simulink library "posAugCoef_cl"  (R2022a)
settings: Solver=VariableStepAuto  StartTime=0.0  StopTime=10.0  RelTol=1e-3
undefined symbols (not defined in the file): aRoll, aYaw, azuSweep, bandGap, bRoll, bYaw, DiscIntNeverNeededParam, elevSet, elevStart, env, fftSwitch, FLIGHTCONTROLLER, fltCtrl, fltCtrlPath, FREQ, hiGainTime, initializeBussesFromBlock, intSat, K_filt, lockTime, orientExitTime, orientLaps, pathEstimCtrl, pathLaps, pthCtrl1, rollAmp, rollFreq, rollPhase, rollPow, thetaIGain, thetaPGain, vhcl, yawAmp, yawFreq, yawPhase
libraries: dspsigops x10, slpidlib x5, firstOrderFilter_ul x3, velocityAngle_ul x2, pathFollowingCtrlAoATurb_cl x1, pathFollowingCtrlAoATurbCoef_cl x1, courseFollowLookAhead_cl x1, ctrlAllocMatrix3CompCoef_cl x1, eulAng2RotMat_ul x1, angleBtw2Vecs_ul x1, vrlib x1, alphaBeta_ul x1
(part 2 of 2)

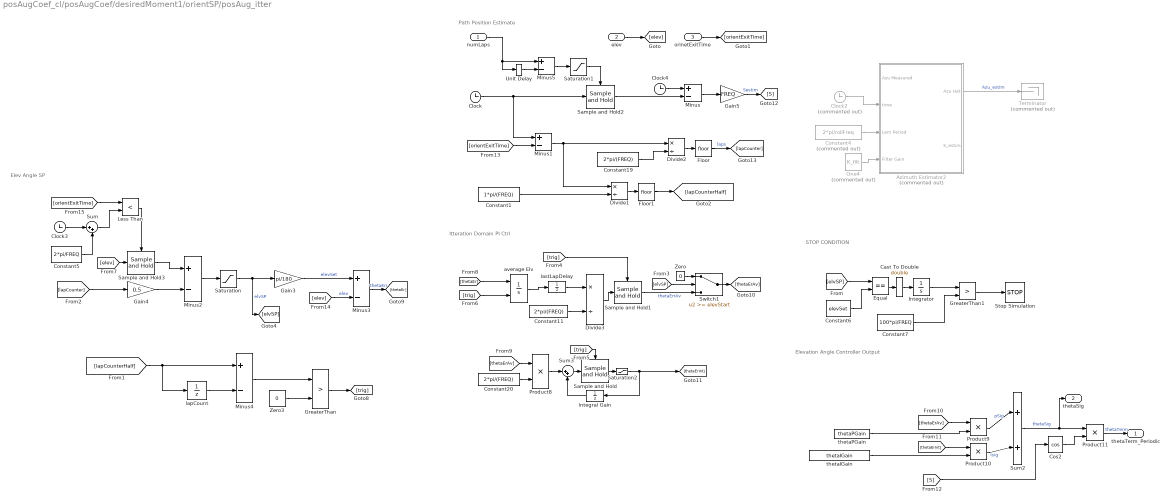
== system posAugCoef_cl/posAugCoef/desiredMoment1/orientSP/posAug_itter ==
  note: STOP CONDITION
  note: Elev Angle SP
  note: Itteration Domain PI Ctrl
  note: Path Position Estimate
  note: Elevation Angle Controller Output
  numLaps : Inport
  elev : Inport  Port=2
  orinetExitTime : Inport  Port=3
  Azimuth Estimator2 : Subsystem  Commented=on
  Cast To Double : DataTypeConversion  OutDataTypeStr=double  SaturateOnIntegerOverflow=off  RndMeth=Floor
  Clock : Clock
  Clock2 : Clock  Commented=on
  Clock3 : Clock
  Clock4 : Clock
  Constant1 : Constant  Value=1*pi/(FREQ)
  Constant11 : Constant  Value=2*pi/(FREQ)
  Constant19 : Constant  Value=2*pi/(FREQ)
  Constant20 : Constant  Value=2*pi/(FREQ)
  Constant4 : Constant  Commented=on  Value=2*pi/rollFreq
  Constant5 : Constant  Value=2*pi/FREQ
  Constant6 : Constant  Value=elevSet
  Constant7 : Constant  Value=100*pi/FREQ
  Cos2 : Trigonometry  Operator=cos
  Divide1 : Product  Inputs=*/
  Divide2 : Product  Inputs=*/
  Divide3 : Product  Inputs=*/
  Equal : RelationalOperator  Operator===  OutDataTypeStr=boolean  RndMeth=Simplest  InputSameDT=off
  Floor : Rounding
  Floor1 : Rounding
  Gain3 : Gain  Gain=pi/180
  Gain4 : Gain  Gain=0.5
  Gain5 : Gain  Gain=FREQ
  GreaterThan : RelationalOperator  Operator=>  OutDataTypeStr=boolean  RndMeth=Simplest  InputSameDT=off
  GreaterThan1 : RelationalOperator  Operator=>  OutDataTypeStr=boolean  RndMeth=Simplest  InputSameDT=off
  Integrator : Integrator
  Less Than : RelationalOperator  Operator=<  OutDataTypeStr=boolean  RndMeth=Simplest  InputSameDT=off
  Minus{,1..5} (6 alike) : Sum  Inputs=+-
  One4 : Constant  Commented=on  Value=K_filt  OutDataTypeStr=Inherit: Inherit via back propagation
  Product{8..11} (4 alike) : Product
  Sample and Hold : dspsigops/Sample and Hold  trig=Rising edge  initCond=0  latchinput=off
  Sample and Hold1 : dspsigops/Sample and Hold  trig=Rising edge  initCond=0  latchinput=off
  Sample and Hold2 : dspsigops/Sample and Hold  trig=Rising edge  initCond=0  latchinput=off
  Sample and Hold3 : dspsigops/Sample and Hold  trig=Rising edge  initCond=elevSet  latchinput=off
  Saturation : Saturate  UpperLimit=elevSet+15  LowerLimit=elevSet
  Saturation1 : Saturate  UpperLimit=pathLaps  LowerLimit=0
  Saturation2 : Saturate  UpperLimit=200  LowerLimit=-200
  Stop Simulation : Stop
  Sum : Sum  Inputs=|++
  Sum2 : Sum  Inputs=|++
  Sum3 : Sum  Inputs=|++
  Switch1 : Switch  Threshold=elevStart  SaturateOnIntegerOverflow=off  InputSameDT=off
  Terminator : Terminator  Commented=on
  Unit Delay : UnitDelay  SampleTime=-1  HasFrameUpgradeWarning=on
  Zero : Constant  Value=0  OutDataTypeStr=Inherit: Inherit via back propagation
  Zero3 : Constant  Value=0  OutDataTypeStr=Inherit: Inherit via back propagation
  average Elv : Integrator  ExternalReset=rising
  integral Gain : UnitDelay  SampleTime=-1  HasFrameUpgradeWarning=on
  lapCount : UnitDelay  SampleTime=-1  HasFrameUpgradeWarning=on
  lastLapDelay : UnitDelay  SampleTime=-1  HasFrameUpgradeWarning=on
  thetaIGain : Constant  Value=thetaIGain
  thetaPGain : Constant  Value=thetaPGain
  thetaTerm_Periodic : Outport
  thetaSig : Outport  Port=2
  wires:
  Sum2/1 -> thetaSig/1, Product11/1  "thetaSig"
  [thetaErAv] -> Product8/1
  lapCount/1 -> Minus4/2
  thetaIGain/1 -> Product10/2
  Product11/1 -> thetaTerm_Periodic/1  "thetaTerm"
  GreaterThan/1 -> [trig]
  thetaPGain/1 -> Product9/2
  [trig] -> average Elv/2
  [thetaErInt] -> Product10/1
  [elev] -> Minus3/2  "elev"
  average Elv/1 -> lastLapDelay/1
  Divide2/1 -> Floor/1
  Zero3/1 -> GreaterThan/2
  Floor/1 -> [lapCounter]  "laps"
  Product10/1 -> Sum2/2  "Isig"
  Product9/1 -> Sum2/1  "pSig"
  Cos2/1 -> Product11/2
  Saturation2/1 -> [thetaErInt], integral Gain/1
  Sample and Hold1/1 -> Switch1/3  "thetaErrAv"
  Product8/1 -> Sum3/1
  [trig] -> Sample and Hold1/Trigger
  [thetaErAv] -> Product9/1
  Constant20/1 -> Product8/2
  Sample and Hold/1 -> Saturation2/1
  integral Gain/1 -> Sum3/2
  Minus1/1 -> Divide1/1, Divide2/1
  Divide3/1 -> Sample and Hold1/1
  Saturation/1 -> [elvSP], Gain3/1  "elvSP"
  Constant11/1 -> Divide3/2
  Gain5/1 -> [S]  "Sestim"
  [trig] -> Sample and Hold/Trigger
  lastLapDelay/1 -> Divide3/1
  Minus3/1 -> [thetaEr]  "thetaErr"
  Minus4/1 -> GreaterThan/1
  [thetaEr] -> average Elv/1
  Sum3/1 -> Sample and Hold/1
  Constant19/1 -> Divide2/2
  Clock/1 -> Minus1/1, Sample and Hold2/1
  elev/1 -> [elev]
  Divide1/1 -> Floor1/1
  Floor1/1 -> [lapCounterHalf]
  Constant1/1 -> Divide1/2
  [lapCounter] -> Gain4/1
  Sample and Hold3/1 -> Minus2/1
  Minus2/1 -> Saturation/1
  Gain3/1 -> Minus3/1  "elevSet"
  numLaps/1 -> Unit Delay/1, Minus5/1
  Unit Delay/1 -> Minus5/2
  [elvSP] -> Switch1/2
  Zero/1 -> Switch1/1
  Switch1/1 -> [thetaErAv]
  Gain4/1 -> Minus2/2
  [orientExitTime] -> Minus1/2
  [lapCounterHalf] -> lapCount/1, Minus4/1
  Constant4/1 -> Azimuth Estimator2/3(Lem Period)
  Clock2/1 -> Azimuth Estimator2/2(time)
  Azimuth Estimator2/1(Azu Hat) -> Terminator/1  "Azu_estim"
  One4/1 -> Azimuth Estimator2/4(Filter Gain)
  [S] -> Cos2/1
  Minus5/1 -> Saturation1/1
  Saturation1/1 -> Sample and Hold2/Trigger
  Clock4/1 -> Minus/1
  [elvSP] -> Equal/1
  Equal/1 -> Cast To Double/1
  Constant6/1 -> Equal/2
  Integrator/1 -> GreaterThan1/1
  Constant7/1 -> GreaterThan1/2
  GreaterThan1/1 -> Stop Simulation/1
  Cast To Double/1 -> Integrator/1
  Minus/1 -> Gain5/1
  [orientExitTime] -> Less Than/1
  Sum/1 -> Less Than/2
  Clock3/1 -> Sum/1
  Constant5/1 -> Sum/2
  Less Than/1 -> Sample and Hold3/Trigger
  [elev] -> Sample and Hold3/1
  orinetExitTime/1 -> [orientExitTime]
  Sample and Hold2/1 -> Minus/2

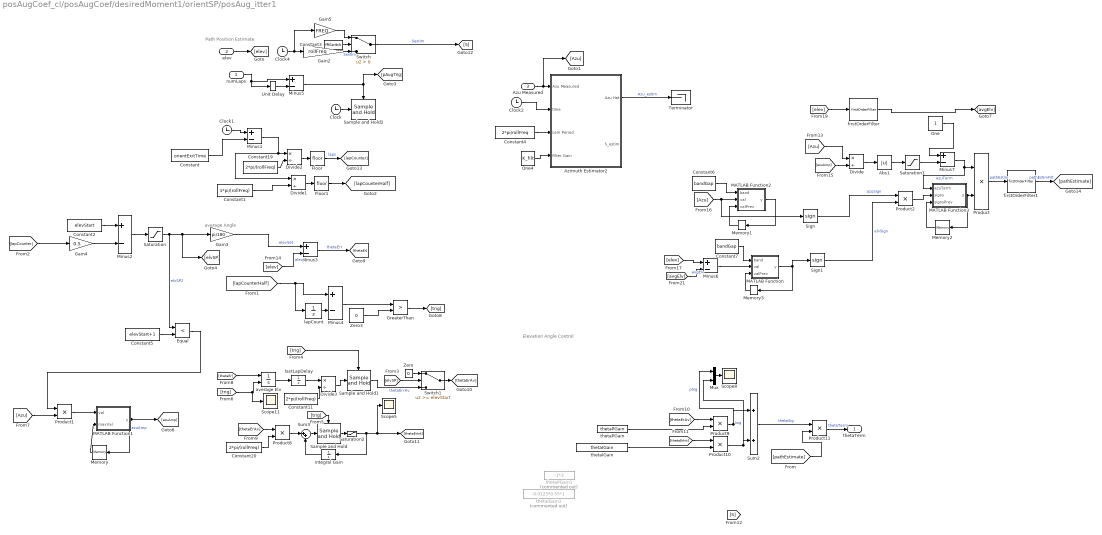
== system posAugCoef_cl/posAugCoef/desiredMoment1/orientSP/posAug_itter1 ==
  note: average Angle
  note: Path Position Estimate
  note: Elevation Angle Control
  numLaps : Inport
  elev : Inport  Port=2
  Azu Measured : Inport  Port=3
  Abs1 : Abs  SaturateOnIntegerOverflow=off
  Azimuth Estimator2 : Subsystem
  Clock{,1..2,4} (4 alike) : Clock
  Constant : Constant  Value=orientExitTime
  Constant1 : Constant  Value=1*pi/(rollFreq)
  Constant11 : Constant  Value=2*pi/(rollFreq)
  Constant19 : Constant  Value=2*pi/(rollFreq)
  Constant2 : Constant  Value=elevStart
  Constant20 : Constant  Value=2*pi/(rollFreq)
  Constant3 : Constant  Value=fftSwitch
  Constant4 : Constant  Value=2*pi/rollFreq
  Constant5 : Constant  Value=elevStart+1
  Constant6 : Constant  Value=bandGap
  Constant7 : Constant  Value=bandGap
  Divide{,1..3} (4 alike) : Product  Inputs=*/
  Equal : RelationalOperator  Operator=<  OutDataTypeStr=boolean  RndMeth=Simplest  InputSameDT=off
  Floor : Rounding
  Floor1 : Rounding
  Gain2 : Gain  Gain=rollFreq
  Gain3 : Gain  Gain=pi/180
  Gain4 : Gain  Gain=0.5
  Gain5 : Gain  Gain=FREQ
  GreaterThan : RelationalOperator  Operator=>  OutDataTypeStr=boolean  RndMeth=Simplest  InputSameDT=off
  MATLAB Function : MATLAB Function  TreatAsAtomicUnit=on
  MATLAB Function1 : MATLAB Function  TreatAsAtomicUnit=on
  MATLAB Function2 : MATLAB Function  TreatAsAtomicUnit=on
  MATLAB Function3 : MATLAB Function  TreatAsAtomicUnit=on
  Memory{,1..3} (4 alike) : Memory
  Minus{1..7} (7 alike) : Sum  Inputs=+-
  Mux : Mux  Inputs=2
  One : Constant  OutDataTypeStr=Inherit: Inherit via back propagation
  One4 : Constant  Value=K_filt  OutDataTypeStr=Inherit: Inherit via back propagation
  Product{,1..2,8..11} (7 alike) : Product
  Sample and Hold : dspsigops/Sample and Hold  trig=Rising edge  initCond=0  latchinput=off
  Sample and Hold1 : dspsigops/Sample and Hold  trig=Rising edge  initCond=0  latchinput=off
  Sample and Hold2 : dspsigops/Sample and Hold  trig=Rising edge  initCond=0  latchinput=off
  Saturation : Saturate  UpperLimit=elevSet+5  LowerLimit=elevSet
  Saturation1 : Saturate  UpperLimit=1  LowerLimit=-1
  Saturation2 : Saturate  UpperLimit=intSat  LowerLimit=-intSat
  Scope11 : Scope
  Scope5 : Scope
  Scope8 : Scope
  Sign : Signum
  Sign1 : Signum
  Sum2 : Sum  Inputs=|++
  Sum3 : Sum  Inputs=|++
  Switch : Switch  Criteria=u2 > Threshold  SaturateOnIntegerOverflow=off  InputSameDT=off
  Switch1 : Switch  Threshold=elevStart  SaturateOnIntegerOverflow=off  InputSameDT=off
  Terminator : Terminator
  Unit Delay : UnitDelay  SampleTime=-1  HasFrameUpgradeWarning=on
  Zero : Constant  Value=0  OutDataTypeStr=Inherit: Inherit via back propagation
  Zero3 : Constant  Value=0  OutDataTypeStr=Inherit: Inherit via back propagation
  average Elv : Integrator  ExternalReset=rising
  firstOrderFilter : firstOrderFilter_ul/firstOrderFilter  tau=elvFilt  ic=0
  firstOrderFilter1 : firstOrderFilter_ul/firstOrderFilter  tau=pathEstimFilt  ic=0
  integral Gain : UnitDelay  SampleTime=-1  HasFrameUpgradeWarning=on
  lapCount : UnitDelay  SampleTime=-1  HasFrameUpgradeWarning=on
  lastLapDelay : UnitDelay  SampleTime=-1  HasFrameUpgradeWarning=on
  thetaIGain : Constant  Value=thetaIGain
  thetaIGain1 : Constant  Commented=on  Value=-0.0125*0.55*1
  thetaPGain : Constant  Value=thetaPGain
  thetaPGain1 : Constant  Commented=on  Value=-1*3
  thetaTerm : Outport
  wires:
  Sum2/1 -> Product11/1  "thetaSig"
  [thetaErAv] -> Product8/1
  lapCount/1 -> Minus4/2
  thetaIGain/1 -> Product10/2
  Product11/1 -> thetaTerm/1  "thetaTerm"
  GreaterThan/1 -> [trig]
  thetaPGain/1 -> Product9/2
  [trig] -> Scope11/1, average Elv/2
  [thetaErInt] -> Product10/1
  [elev] -> Minus3/2  "elev"
  average Elv/1 -> lastLapDelay/1
  Divide2/1 -> Floor/1
  Zero3/1 -> GreaterThan/2
  Floor/1 -> [lapCounter]  "laps"
  Product10/1 -> Mux/2, Sum2/2  "Isig"
  Mux/1 -> Scope8/1
  Product9/1 -> Mux/1, Sum2/1  "pSig"
  Saturation2/1 -> Scope5/1, [thetaErInt], integral Gain/1
  Sample and Hold1/1 -> Switch1/3  "thetaErrAv"
  Product8/1 -> Sum3/1
  [trig] -> Sample and Hold1/Trigger
  [thetaErAv] -> Product9/1
  Constant20/1 -> Product8/2
  Sample and Hold/1 -> Saturation2/1
  integral Gain/1 -> Sum3/2
  Minus1/1 -> Divide1/1, Divide2/1
  Divide3/1 -> Sample and Hold1/1
  Clock4/1 -> Gain5/1, Gain2/1
  Saturation/1 -> Equal/1, [elvSP], Gain3/1  "elvSP2"
  Constant11/1 -> Divide3/2
  Switch/1 -> [S]  "Sestim"
  [trig] -> Sample and Hold/Trigger
  lastLapDelay/1 -> Divide3/1
  Minus3/1 -> [thetaEr]  "thetaErr"
  Minus4/1 -> GreaterThan/1
  [thetaEr] -> average Elv/1
  Sum3/1 -> Sample and Hold/1
  Constant19/1 -> Divide2/2
  Clock1/1 -> Minus1/1
  elev/1 -> [elev]
  Minus5/1 -> [pAugTrig], Sample and Hold2/Trigger
  Clock/1 -> Sample and Hold2/1
  Divide1/1 -> Floor1/1
  Floor1/1 -> [lapCounterHalf]
  Constant1/1 -> Divide1/2
  [lapCounter] -> Gain4/1
  Constant2/1 -> Minus2/1
  Minus2/1 -> Saturation/1
  Gain3/1 -> Minus3/1  "elevSet"
  numLaps/1 -> Unit Delay/1, Minus5/1
  Unit Delay/1 -> Minus5/2
  [elvSP] -> Switch1/2
  Zero/1 -> Switch1/1
  Switch1/1 -> [thetaErAv]
  Gain4/1 -> Minus2/2
  Constant/1 -> Minus1/2
  [lapCounterHalf] -> lapCount/1, Minus4/1
  Constant3/1 -> Switch/2
  Gain2/1 -> Switch/3  "Sestim"
  Gain5/1 -> Switch/1
  Constant4/1 -> Azimuth Estimator2/3(Lem Period)
  Clock2/1 -> Azimuth Estimator2/2(time)
  Azimuth Estimator2/1(Azu Hat) -> Terminator/1  "Azu_estim"
  One4/1 -> Azimuth Estimator2/4(Filter Gain)
  Azu Measured/1 -> [Azu], Azimuth Estimator2/1(Azu Measured)
  Equal/1 -> Product1/1
  Memory/1 -> MATLAB Function1/2(maxVal)
  Product1/1 -> MATLAB Function1/1(val)
  MATLAB Function1/1(y) -> Memory/1, [azuAmp]  "azuAmp"
  Constant5/1 -> Equal/2
  [Azu] -> Product1/2
  Memory2/1 -> MATLAB Function3/3(signsPrev)
  MATLAB Function3/1(y) -> Memory2/1, Product/2
  Sign1/1 -> Product2/2  "elvSign"
  [Azu] -> Sign/1, MATLAB Function2/2(val)
  MATLAB Function/1(y) -> Memory3/1, Sign1/1
  [elev] -> Minus6/1
  Abs1/1 -> Saturation1/1
  firstOrderFilter1/1 -> [pathEstimate]  "pathEstimFilt"
  Minus7/1 -> MATLAB Function3/1(azuTerm), Product/1  "azuTerm"
  Memory3/1 -> MATLAB Function/3(valPrev)
  One/1 -> Minus7/1
  [elev] -> firstOrderFilter/1
  Constant6/1 -> MATLAB Function2/1(band)
  Product/1 -> firstOrderFilter1/1  "pathEstim"
  Saturation1/1 -> Minus7/2
  firstOrderFilter/1 -> [avgElv]
  Constant7/1 -> MATLAB Function/1(band)
  MATLAB Function2/1(y) -> Memory1/1
  Minus6/1 -> MATLAB Function/2(val)
  Sign/1 -> Product2/1  "azuSign"
  Memory1/1 -> MATLAB Function2/3(valPrev)
  [Azu] -> Divide/1
  [avgElv] -> Minus6/2  "avgElv"
  Divide/1 -> Abs1/1
  Product2/1 -> MATLAB Function3/2(signs)
  [azuAmp] -> Divide/2
  [pathEstimate] -> Product11/2

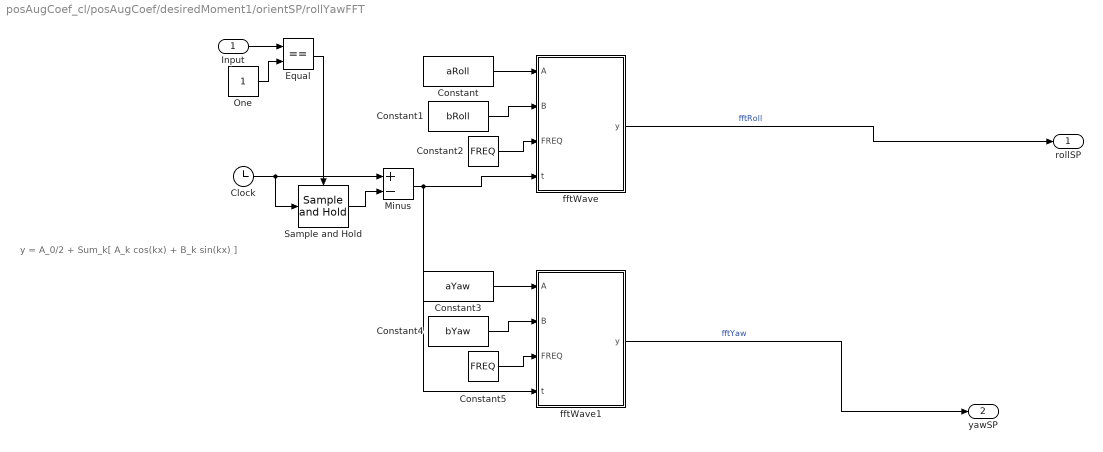
== system posAugCoef_cl/posAugCoef/desiredMoment1/orientSP/rollYawFFT ==
  note: y = A_0/2 + Sum_k[ A_k cos(kx) + B_k sin(kx) ]
  Input : Inport
  Clock : Clock
  Constant : Constant  Value=aRoll
  Constant1 : Constant  Value=bRoll
  Constant2 : Constant  Value=FREQ
  Constant3 : Constant  Value=aYaw
  Constant4 : Constant  Value=bYaw
  Constant5 : Constant  Value=FREQ
  Equal : RelationalOperator  Operator===  OutDataTypeStr=boolean  RndMeth=Simplest  InputSameDT=off
  Minus : Sum  Inputs=+-
  One : Constant  OutDataTypeStr=Inherit: Inherit via back propagation
  Sample and Hold : dspsigops/Sample and Hold  trig=Rising edge  initCond=0  latchinput=off
  fftWave : MATLAB Function  TreatAsAtomicUnit=on
  fftWave1 : MATLAB Function  TreatAsAtomicUnit=on
  rollSP : Outport
  yawSP : Outport  Port=2
  wires:
  Constant2/1 -> fftWave/3(FREQ)
  Constant1/1 -> fftWave/2(B)
  Constant/1 -> fftWave/1(A)
  Constant4/1 -> fftWave1/2(B)
  Constant5/1 -> fftWave1/3(FREQ)
  Constant3/1 -> fftWave1/1(A)
  Minus/1 -> fftWave/4(t), fftWave1/4(t)
  fftWave1/1(y) -> yawSP/1  "fftYaw"
  fftWave/1(y) -> rollSP/1  "fftRoll"
  Input/1 -> Equal/1
  One/1 -> Equal/2
  Equal/1 -> Sample and Hold/Trigger
  Clock/1 -> Minus/1, Sample and Hold/1
  Sample and Hold/1 -> Minus/2

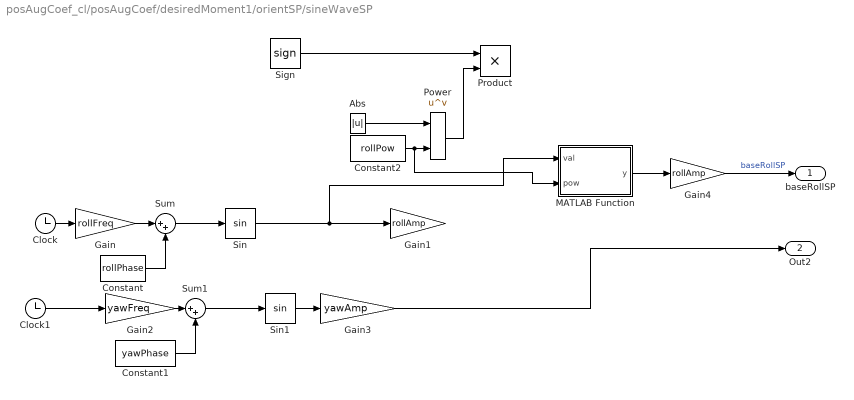
== system posAugCoef_cl/posAugCoef/desiredMoment1/orientSP/sineWaveSP ==
  Abs : Abs  SaturateOnIntegerOverflow=off
  Clock : Clock
  Clock1 : Clock
  Constant : Constant  Value=rollPhase
  Constant1 : Constant  Value=yawPhase
  Constant2 : Constant  Value=rollPow
  Gain : Gain  Gain=rollFreq
  Gain1 : Gain  Gain=rollAmp
  Gain2 : Gain  Gain=yawFreq
  Gain3 : Gain  Gain=yawAmp
  Gain4 : Gain  Gain=rollAmp
  MATLAB Function : MATLAB Function  TreatAsAtomicUnit=on
  Power : Math  Operator=pow
  Product : Product
  Sign : Signum
  Sin : Trigonometry
  Sin1 : Trigonometry
  Sum : Sum  Inputs=|++
  Sum1 : Sum  Inputs=|++
  baseRollSP : Outport
  Out2 : Outport  Port=2
  wires:
  Sum/1 -> Sin/1
  Sum1/1 -> Sin1/1
  Constant/1 -> Sum/2
  Gain/1 -> Sum/1
  Gain2/1 -> Sum1/1
  Constant1/1 -> Sum1/2
  Sin1/1 -> Gain3/1
  Clock/1 -> Gain/1
  Clock1/1 -> Gain2/1
  Gain3/1 -> Out2/1
  Sin/1 -> MATLAB Function/1(val), Gain1/1
  Sign/1 -> Product/1
  Constant2/1 -> MATLAB Function/2(pow), Power/2
  Abs/1 -> Power/1
  Power/1 -> Product/2
  MATLAB Function/1(y) -> Gain4/1
  Gain4/1 -> baseRollSP/1  "baseRollSP"

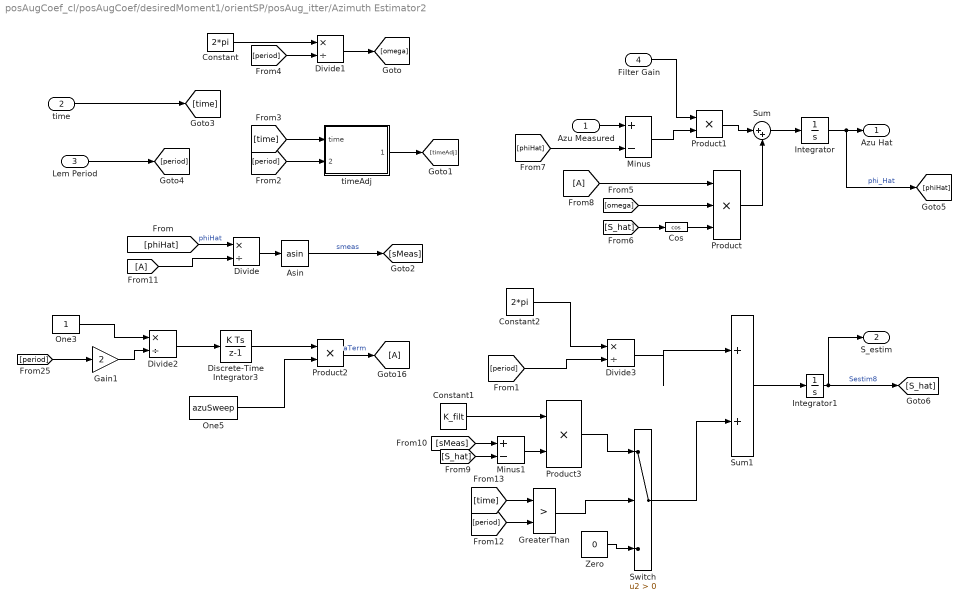
== system posAugCoef_cl/posAugCoef/desiredMoment1/orientSP/posAug_itter/Azimuth Estimator2 ==
  Azu Measured : Inport
  time : Inport  Port=2
  Lem Period : Inport  Port=3
  Filter Gain : Inport  Port=4
  Asin : Trigonometry  Operator=asin
  Constant : Constant  Value=2*pi  OutDataTypeStr=single
  Constant1 : Constant  Value=K_filt
  Constant2 : Constant  Value=2*pi
  Cos : Trigonometry  Operator=cos
  Discrete-Time Integrator3 : DiscreteIntegrator  SampleTime=-1  LimitOutput=on  UpperSaturationLimit=1  LowerSaturationLimit=0  ICPrevOutput=DiscIntNeverNeededParam  ICPrevScaledInput=DiscIntNeverNeededParam
  Divide{,1..3} (4 alike) : Product  Inputs=*/
  From11 : From
  From8 : From
  Gain1 : Gain  Gain=2
  Goto16 : Goto
  GreaterThan : RelationalOperator  Operator=>  OutDataTypeStr=boolean  RndMeth=Simplest  InputSameDT=off
  Integrator : Integrator
  Integrator1 : Integrator
  Minus : Sum  Inputs=+-
  Minus1 : Sum  Inputs=+-
  One3 : Constant  OutDataTypeStr=single
  One5 : Constant  Value=azuSweep  OutDataTypeStr=Inherit: Inherit via back propagation
  Product : Product  Inputs=3
  Product1 : Product
  Product2 : Product
  Product3 : Product
  Sum : Sum  Inputs=|++
  Sum1 : Sum  Inputs=|++
  Switch : Switch  Criteria=u2 > Threshold  SaturateOnIntegerOverflow=off  InputSameDT=off
  Zero : Constant  Value=0  OutDataTypeStr=Inherit: Inherit via back propagation
  timeAdj : MATLAB Function  TreatAsAtomicUnit=on
  Azu Hat : Outport
  S_estim : Outport  Port=2
  wires:
  timeAdj/1(timeAdj) -> [timeAdj]
  [period] -> timeAdj/2(Lem_Period)
  [time] -> timeAdj/1(time)
  [period] -> Divide1/2
  Divide1/1 -> [omega]
  Minus/1 -> Product1/2
  Azu Measured/1 -> Minus/1
  Sum/1 -> Integrator/1
  Product1/1 -> Sum/1
  From8/1 -> Product/1
  [omega] -> Product/2
  [S_hat] -> Cos/1
  Cos/1 -> Product/3
  Product/1 -> Sum/2
  Integrator/1 -> [phiHat], Azu Hat/1  "phi_Hat"
  [phiHat] -> Minus/2
  Constant/1 -> Divide1/1
  Filter Gain/1 -> Product1/1
  Lem Period/1 -> [period]
  time/1 -> [time]
  Product2/1 -> Goto16/1  "aTerm"
  One3/1 -> Divide2/1
  Gain1/1 -> Divide2/2
  [period] -> Gain1/1
  Discrete-Time Integrator3/1 -> Product2/1
  Divide2/1 -> Discrete-Time Integrator3/1
  One5/1 -> Product2/2
  Sum1/1 -> Integrator1/1
  [sMeas] -> Minus1/1
  Product3/1 -> Switch/1
  Constant1/1 -> Product3/1
  [S_hat] -> Minus1/2
  Divide3/1 -> Sum1/1
  Minus1/1 -> Product3/2
  [period] -> Divide3/2
  Constant2/1 -> Divide3/1
  Asin/1 -> [sMeas]  "smeas"
  [phiHat] -> Divide/1  "phiHat"
  From11/1 -> Divide/2
  Divide/1 -> Asin/1
  Integrator1/1 -> [S_hat], S_estim/1  "Sestim8"
  Switch/1 -> Sum1/2
  Zero/1 -> Switch/3
  [time] -> GreaterThan/1
  [period] -> GreaterThan/2
  GreaterThan/1 -> Switch/2

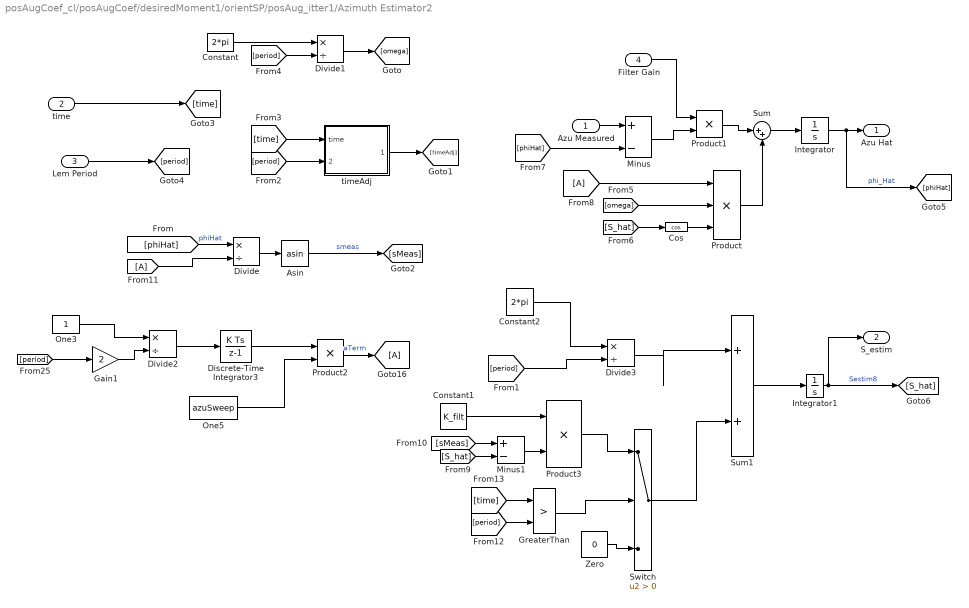
== system posAugCoef_cl/posAugCoef/desiredMoment1/orientSP/posAug_itter1/Azimuth Estimator2 ==
  Azu Measured : Inport
  time : Inport  Port=2
  Lem Period : Inport  Port=3
  Filter Gain : Inport  Port=4
  Asin : Trigonometry  Operator=asin
  Constant : Constant  Value=2*pi  OutDataTypeStr=single
  Constant1 : Constant  Value=K_filt
  Constant2 : Constant  Value=2*pi
  Cos : Trigonometry  Operator=cos
  Discrete-Time Integrator3 : DiscreteIntegrator  SampleTime=-1  LimitOutput=on  UpperSaturationLimit=1  LowerSaturationLimit=0  ICPrevOutput=DiscIntNeverNeededParam  ICPrevScaledInput=DiscIntNeverNeededParam
  Divide{,1..3} (4 alike) : Product  Inputs=*/
  From11 : From
  From8 : From
  Gain1 : Gain  Gain=2
  Goto16 : Goto
  GreaterThan : RelationalOperator  Operator=>  OutDataTypeStr=boolean  RndMeth=Simplest  InputSameDT=off
  Integrator : Integrator
  Integrator1 : Integrator
  Minus : Sum  Inputs=+-
  Minus1 : Sum  Inputs=+-
  One3 : Constant  OutDataTypeStr=single
  One5 : Constant  Value=azuSweep  OutDataTypeStr=Inherit: Inherit via back propagation
  Product : Product  Inputs=3
  Product1 : Product
  Product2 : Product
  Product3 : Product
  Sum : Sum  Inputs=|++
  Sum1 : Sum  Inputs=|++
  Switch : Switch  Criteria=u2 > Threshold  SaturateOnIntegerOverflow=off  InputSameDT=off
  Zero : Constant  Value=0  OutDataTypeStr=Inherit: Inherit via back propagation
  timeAdj : MATLAB Function  TreatAsAtomicUnit=on
  Azu Hat : Outport
  S_estim : Outport  Port=2
  wires:
  timeAdj/1(timeAdj) -> [timeAdj]
  [period] -> timeAdj/2(Lem_Period)
  [time] -> timeAdj/1(time)
  [period] -> Divide1/2
  Divide1/1 -> [omega]
  Minus/1 -> Product1/2
  Azu Measured/1 -> Minus/1
  Sum/1 -> Integrator/1
  Product1/1 -> Sum/1
  From8/1 -> Product/1
  [omega] -> Product/2
  [S_hat] -> Cos/1
  Cos/1 -> Product/3
  Product/1 -> Sum/2
  Integrator/1 -> [phiHat], Azu Hat/1  "phi_Hat"
  [phiHat] -> Minus/2
  Constant/1 -> Divide1/1
  Filter Gain/1 -> Product1/1
  Lem Period/1 -> [period]
  time/1 -> [time]
  Product2/1 -> Goto16/1  "aTerm"
  One3/1 -> Divide2/1
  Gain1/1 -> Divide2/2
  [period] -> Gain1/1
  Discrete-Time Integrator3/1 -> Product2/1
  Divide2/1 -> Discrete-Time Integrator3/1
  One5/1 -> Product2/2
  Sum1/1 -> Integrator1/1
  [sMeas] -> Minus1/1
  Product3/1 -> Switch/1
  Constant1/1 -> Product3/1
  [S_hat] -> Minus1/2
  Divide3/1 -> Sum1/1
  Minus1/1 -> Product3/2
  [period] -> Divide3/2
  Constant2/1 -> Divide3/1
  Asin/1 -> [sMeas]  "smeas"
  [phiHat] -> Divide/1  "phiHat"
  From11/1 -> Divide/2
  Divide/1 -> Asin/1
  Integrator1/1 -> [S_hat], S_estim/1  "Sestim8"
  Switch/1 -> Sum1/2
  Zero/1 -> Switch/3
  [time] -> GreaterThan/1
  [period] -> GreaterThan/2
  GreaterThan/1 -> Switch/2

== matlab function posAugCoef_cl/posAugCoef/desiredMoment1/orientSP/rollYawFFT/fftWave1 ==
  data: A input; y output; B input; FREQ input; t input
function y = fcn(A,B,FREQ,t)
% 
% A_0=A(1);
% 
% y = A_0/2;
% 
% for k=1:numel(B)
% y=y+ A(k+1)*cos(k*t*FREQ) + B(k)*sin(k*t*FREQ);
% end
y=Fseriesval2(A,B,pi+2*pi*t./(2*pi/FREQ));



end

== matlab function posAugCoef_cl/posAugCoef/desiredMoment1/orientSP/rollYawFFT/fftWave ==
  data: A input; y output; B input; FREQ input; t input
function y = fcn(A,B,FREQ,t)

% A_0=A(1);
% 
% y = A_0/2;
% 
% for k=1:numel(B)
% y=y+ A(k+1)*cos(k*t*FREQ) + B(k)*sin(k*t*FREQ);
% end
% 

y=Fseriesval2(A,B,pi+2*pi*t./(2*pi/FREQ));


end

== matlab function posAugCoef_cl/posAugCoef/desiredMoment1/MATLAB Function1 ==
  data: rollSP input; y output; maxSP input
function y = fcn(rollSP, maxSP)

if abs(rollSP)>abs(maxSP)
    y=abs(rollSP);
else
    y=maxSP;
end

== matlab function posAugCoef_cl/posAugCoef/desiredMoment1/orientSP/posAug_itter1/Azimuth Estimator2/timeAdj ==
  data: time input; timeAdj output; Lem_Period input
function timeAdj = fcn(time,Lem_Period)
timeAdj=time-floor(time/Lem_Period).*Lem_Period;
end

== matlab function posAugCoef_cl/posAugCoef/desiredMoment1/orientSP/posAug_itter1/MATLAB Function1 ==
  data: val input; y output; maxVal input
function y = fcn(val, maxVal)

if abs(val)>abs(maxVal)
    y=abs(val);
else
    y=maxVal;
end

== matlab function posAugCoef_cl/posAugCoef/desiredMoment1/orientSP/posAug_itter1/MATLAB Function ==
  data: band input; y output; val input; valPrev input
function y = hyster(band,val,valPrev)

if abs(val)<band
    y=valPrev;
else
    y=val;
end

== matlab function posAugCoef_cl/posAugCoef/desiredMoment1/orientSP/posAug_itter1/MATLAB Function2 ==
  data: band input; y output; val input; valPrev input
function y = hyster(band,val,valPrev)

if abs(val)<band
    y=valPrev;
else
    y=val;
end

== matlab function posAugCoef_cl/posAugCoef/desiredMoment1/orientSP/posAug_itter1/MATLAB Function3 ==
  data: azuTerm input; y output; signs input; signsPrev input
function y = fcn(azuTerm,signs,signsPrev)


if abs(azuTerm)>0.5
    y=signsPrev;
else
    y=signs;
end

== matlab function posAugCoef_cl/posAugCoef/desiredMoment1/orientSP/sineWaveSP/MATLAB Function ==
  data: val input; y output; pow input
function y = fcn(val,pow)

y = sign(val)*sqrt(val^2)^pow;
end

== matlab function posAugCoef_cl/posAugCoef/desiredMoment1/orientSP/posAug_itter/Azimuth Estimator2/timeAdj ==
  data: time input; timeAdj output; Lem_Period input
function timeAdj = fcn(time,Lem_Period)
timeAdj=time-floor(time/Lem_Period).*Lem_Period;
end
